simulink model "Trabalho1_Jesse_Beatriz_simulink"  (R2016a)
settings: Solver=VariableStepAuto  StartTime=0.0  StopTime=30  RelTol=1e-3
libraries: simulink x9
settings Model: Creator=jessa  LastModifiedBy=jessa

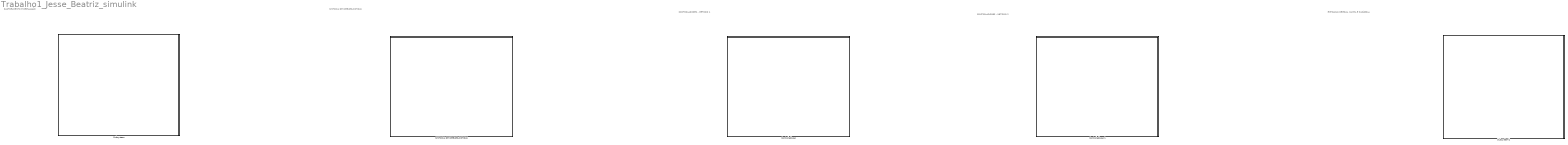
== system Trabalho1_Jesse_Beatriz_simulink ==
  note: CONTROLADORES - METODO 1
  note: SINTONIA DE ZIEGLER-NICHOLS
  note: CONTROLADORES - METODO 2
  note: RASTREAMENTO E REGULAÇÃO
  note: ENTRADAS DEGRAU, RAMPA E PARÁBOLA
  "Controladores " : Subsystem
  Controladores 1 : Subsystem
  SINTONIA DE ZIEGLER-NICHOLS : Subsystem
  Subsystem : Subsystem
  Subsystem1 : Subsystem

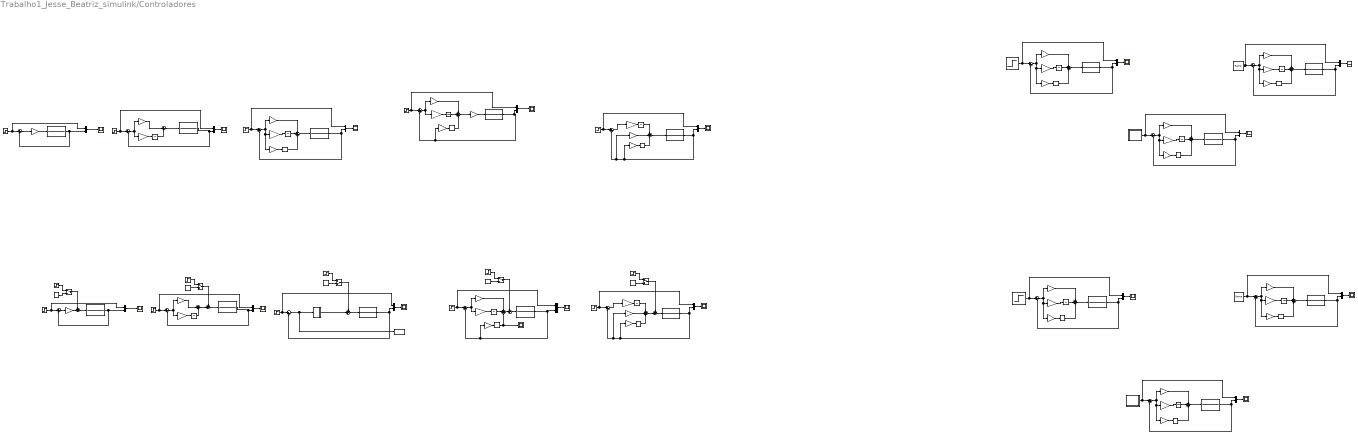
== system Trabalho1_Jesse_Beatriz_simulink/Controladores  ==
  note: E(s)
  note: U(s)
  note: PROPORCIONAL (P)
  note: PROPORCIONAL - INTEGRAL (PI)
  note: PROPORCIONAL - INTEGRAL - DERIVATIVO (PID)
  note: METODO 1
  note: PROPORCIONAL (P)
  note: PROPORCIONAL - INTEGRAL (PI)
  note: PROPORCIONAL - INTEGRAL - DERIVATIVO (PID)
  note: Controlador Sintonizado
  note: E(s)
  note: E(s)
  note: U(s)
  note: PI-D
  note: I-PD
  note: E(s)
  note: E(s)
  note: PI-D
  note: I-PD
  note: DEGRAU
  note: RAMPA
  note: PARABOLA
  note: ENTRADAS DEGRAU, RAMPA E PARÁBOLA
  note: E(s)
  note: U(s)
  note: E(s)
  note: U(s)
  note: E(s)
  note: U(s)
  note: E(s)
  note: U(s)
  note: E(s)
  note: U(s)
  note: E(s)
  note: U(s)
  note: DEGRAU
  note: RAMPA
  note: PARABOLA
  Constant{,1..4} (5 alike) : Constant  Value=0
  Derivative{,2..11} (11 alike) : Derivative
  Entrada Parabola Unitaria : Subsystem
  Entrada Parabola Unitaria1 : Subsystem
  Gain : Gain  Gain=8.0185
  Gain1 : Gain  Gain=6
  Integrator{,1..2,4..13} (13 alike) : Integrator
  Ki : Gain  Gain=10.8304
  Ki{1,8,14,16,18} (5 alike) : Gain  Gain=24.0676
  Ki{10,20,22,24} (4 alike) : Gain  Gain=5
  Ki{3,11,13,21,23,25} (6 alike) : Gain  Gain=2
  Ki12 : Gain  Gain=9
  Ki{2,9,15,17,19} (5 alike) : Gain  Gain=0.9617
  Ki6 : Gain  Gain=2.5013
  Ki7 : Gain  Gain=0.099
  Kp : Gain  Gain=7.2167
  Kp{1,5,8..11} (6 alike) : Gain  Gain=9.6222
  Kp{6,12..14} (4 alike) : Gain  Gain=12
  Kp2 : Gain  Gain=4
  Kp4 : Gain
  Kp7 : Gain  Gain=5
  Manual Switch{,1,3..4} (4 alike) : ManualSwitch
  Manual Switch2 : ManualSwitch  CurrentSetting=0
  Mux{1..16} (16 alike) : Mux  Inputs=2
  PID_Sintonizado : Subsystem
  Ramp : simulink/Sources/Ramp  slope=1  start=0  X0=0
  Ramp1 : simulink/Sources/Ramp  slope=1  start=0  X0=0
  Scope{1..16,18} (17 alike) : Scope
  Step{1..2,4..5,7..8,10..11,15} (9 alike) : Step  Time=0  SampleTime=0
  Step{12..14,16..17} (5 alike) : Step  Time=10  After=-1  SampleTime=0
  Step3 : Step  SampleTime=0
  Step6 : Step  SampleTime=0
  Step9 : Step  SampleTime=0
  Sum{1..2,4,6..7,9,11,13,15,17,19,21,23,26,28,30} (16 alike) : Sum  Inputs=|+-
  Sum12 : Sum  Inputs=++-
  Sum14 : Sum  Inputs=+--
  Sum16 : Sum  Inputs=++-
  Sum18 : Sum  Inputs=+--
  Sum{5,20,22,24..25,27,29} (7 alike) : Sum  Inputs=+++
  Sum3 : Sum  Inputs=|++
  Sum{31..35} (5 alike) : Sum  Inputs=++|
  Sum8 : Sum  Inputs=|++
  To Workspace : ToWorkspace  VariableName=Erro_PID  SampleTime=-1
  Transfer Fcn{1..16} (16 alike) : TransferFcn  Numerator=[45]  Denominator=[1 15 59 45]
  wires:
  Sum1/1 -> Gain/1
  Mux1/1 -> Scope1/1
  Transfer Fcn1/1 -> Sum1/2, Mux1/2
  Step1/1 -> Sum1/1, Mux1/1
  Gain/1 -> Transfer Fcn1/1
  Sum2/1 -> Ki/1, Kp/1
  Mux2/1 -> Scope2/1
  Transfer Fcn2/1 -> Mux2/2, Sum2/2
  Step2/1 -> Sum2/1, Mux2/1
  Kp/1 -> Sum3/1
  Sum3/1 -> Transfer Fcn2/1
  Ki/1 -> Integrator/1
  Integrator/1 -> Sum3/2
  Sum4/1 -> Kp1/1, Ki2/1, Ki1/1
  Mux3/1 -> Scope3/1
  Transfer Fcn3/1 -> Mux3/2, Sum4/2
  Step3/1 -> Mux3/1, Sum4/1
  Kp1/1 -> Sum5/1
  Sum5/1 -> Transfer Fcn3/1
  Ki1/1 -> Integrator1/1
  Integrator1/1 -> Sum5/2
  Ki2/1 -> Derivative/1
  Derivative/1 -> Sum5/3
  Sum6/1 -> Gain1/1
  Mux4/1 -> Scope4/1
  Transfer Fcn4/1 -> Mux4/2, Sum6/2
  Step4/1 -> Mux4/1, Sum6/1
  Sum7/1 -> Kp2/1, Ki3/1
  Mux5/1 -> Scope5/1
  Transfer Fcn5/1 -> Sum7/2, Mux5/2
  Step5/1 -> Mux5/1, Sum7/1
  Kp2/1 -> Sum8/1
  Ki3/1 -> Integrator2/1
  Integrator2/1 -> Sum8/2
  Mux6/1 -> Scope6/1
  Transfer Fcn6/1 -> Sum9/2, Mux6/2
  Step6/1 -> Mux6/1, Sum9/1
  Sum11/1 -> Ki6/1, Kp4/1
  Mux7/1 -> Scope7/1
  Transfer Fcn7/1 -> Ki7/1, Sum11/2, Mux7/2
  Step7/1 -> Sum11/1, Mux7/1
  Kp4/1 -> Sum12/1
  Ki6/1 -> Integrator4/1
  Integrator4/1 -> Sum12/2
  Ki7/1 -> Derivative2/1
  Derivative2/1 -> Sum12/3
  Sum13/1 -> Ki8/1
  Mux8/1 -> Scope8/1
  Transfer Fcn8/1 -> Mux8/2, Ki9/1, Kp5/1, Sum13/2
  Step8/1 -> Mux8/1, Sum13/1
  Sum14/1 -> Transfer Fcn8/1
  Ki8/1 -> Integrator5/1
  Ki9/1 -> Derivative3/1
  Derivative3/1 -> Sum14/3
  Kp5/1 -> Sum14/2
  Integrator5/1 -> Sum14/1
  Sum15/1 -> Kp6/1, Ki10/1
  Mux9/1 -> Scope9/1
  Transfer Fcn9/1 -> Mux9/2, Sum15/2, Ki11/1
  Step9/1 -> Mux9/1, Sum15/1
  Kp6/1 -> Sum16/1
  Ki10/1 -> Integrator6/1
  Integrator6/1 -> Sum16/2
  Ki11/1 -> Derivative4/1
  Sum17/1 -> Ki12/1
  Mux10/1 -> Scope10/1
  Transfer Fcn10/1 -> Sum17/2, Kp7/1, Ki13/1, Mux10/2
  Step10/1 -> Sum17/1, Mux10/1
  Ki12/1 -> Integrator7/1
  Ki13/1 -> Derivative5/1
  Derivative5/1 -> Sum18/3
  Kp7/1 -> Sum18/2
  Integrator7/1 -> Sum18/1
  Kp8/1 -> Transfer Fcn7/1
  Sum12/1 -> Kp8/1
  Sum19/1 -> Kp9/1, Ki15/1, Ki14/1
  Mux11/1 -> Scope11/1
  Transfer Fcn11/1 -> Mux11/2, Sum19/2
  Step11/1 -> Mux11/1, Sum19/1
  Kp9/1 -> Sum20/1
  Sum20/1 -> Transfer Fcn11/1
  Ki14/1 -> Integrator8/1
  Integrator8/1 -> Sum20/2
  Ki15/1 -> Derivative6/1
  Derivative6/1 -> Sum20/3
  Sum21/1 -> Kp10/1, Ki17/1, Ki16/1
  Mux12/1 -> Scope12/1
  Transfer Fcn12/1 -> Mux12/2, Sum21/2
  Entrada Parabola Unitaria/1(Out1) -> Mux12/1, Sum21/1
  Kp10/1 -> Sum22/1
  Sum22/1 -> Transfer Fcn12/1
  Ki16/1 -> Integrator9/1
  Integrator9/1 -> Sum22/2
  Ki17/1 -> Derivative7/1
  Derivative7/1 -> Sum22/3
  Sum23/1 -> Kp11/1, Ki19/1, Ki18/1
  Mux13/1 -> Scope13/1
  Transfer Fcn13/1 -> Mux13/2, Sum23/2
  Ramp/1 -> Mux13/1, Sum23/1
  Kp11/1 -> Sum24/1
  Sum24/1 -> Transfer Fcn13/1
  Ki18/1 -> Integrator10/1
  Integrator10/1 -> Sum24/2
  Ki19/1 -> Derivative8/1
  Derivative8/1 -> Sum24/3
  Sum26/1 -> Ki20/1, Ki21/1, Kp12/1
  Mux14/1 -> Scope14/1
  Transfer Fcn14/1 -> Sum26/2, Mux14/2
  Step15/1 -> Sum26/1, Mux14/1
  Kp12/1 -> Sum25/1
  Sum25/1 -> Transfer Fcn14/1
  Ki20/1 -> Integrator11/1
  Integrator11/1 -> Sum25/2
  Ki21/1 -> Derivative9/1
  Derivative9/1 -> Sum25/3
  Sum28/1 -> Ki23/1, Ki22/1, Kp13/1
  Mux15/1 -> Scope15/1
  Transfer Fcn15/1 -> Sum28/2, Mux15/2
  Ramp1/1 -> Sum28/1, Mux15/1
  Kp13/1 -> Sum27/1
  Sum27/1 -> Transfer Fcn15/1
  Ki22/1 -> Integrator12/1
  Integrator12/1 -> Sum27/2
  Ki23/1 -> Derivative10/1
  Derivative10/1 -> Sum27/3
  Sum30/1 -> Ki24/1, Ki25/1, Kp14/1
  Mux16/1 -> Scope16/1
  Transfer Fcn16/1 -> Sum30/2, Mux16/2
  Entrada Parabola Unitaria1/1(Out1) -> Sum30/1, Mux16/1
  Kp14/1 -> Sum29/1
  Sum29/1 -> Transfer Fcn16/1
  Ki24/1 -> Integrator13/1
  Integrator13/1 -> Sum29/2
  Ki25/1 -> Derivative11/1
  Derivative11/1 -> Sum29/3
  Gain1/1 -> Sum31/2
  Sum31/1 -> Transfer Fcn4/1
  Step12/1 -> Manual Switch/1
  Manual Switch/1 -> Sum31/1
  Step13/1 -> Manual Switch1/1
  Manual Switch1/1 -> Sum32/1
  Sum8/1 -> Sum32/2
  Sum32/1 -> Transfer Fcn5/1
  Step14/1 -> Manual Switch2/1
  Manual Switch2/1 -> Sum33/1
  Sum33/1 -> Transfer Fcn6/1
  Step16/1 -> Manual Switch3/1
  Manual Switch3/1 -> Sum34/1
  Step17/1 -> Manual Switch4/1
  Manual Switch4/1 -> Sum35/1
  Sum16/1 -> Sum34/2
  Sum34/1 -> Transfer Fcn9/1
  Sum18/1 -> Sum35/2
  Sum35/1 -> Transfer Fcn10/1
  Constant/1 -> Manual Switch/2
  Constant1/1 -> Manual Switch1/2
  Constant2/1 -> Manual Switch2/2
  Constant3/1 -> Manual Switch3/2
  Constant4/1 -> Manual Switch4/2
  Derivative4/1 -> Scope18/1, Sum16/3
  PID_Sintonizado/1(Out1) -> Sum33/2
  Sum9/1 -> To Workspace/1, PID_Sintonizado/1(In1)

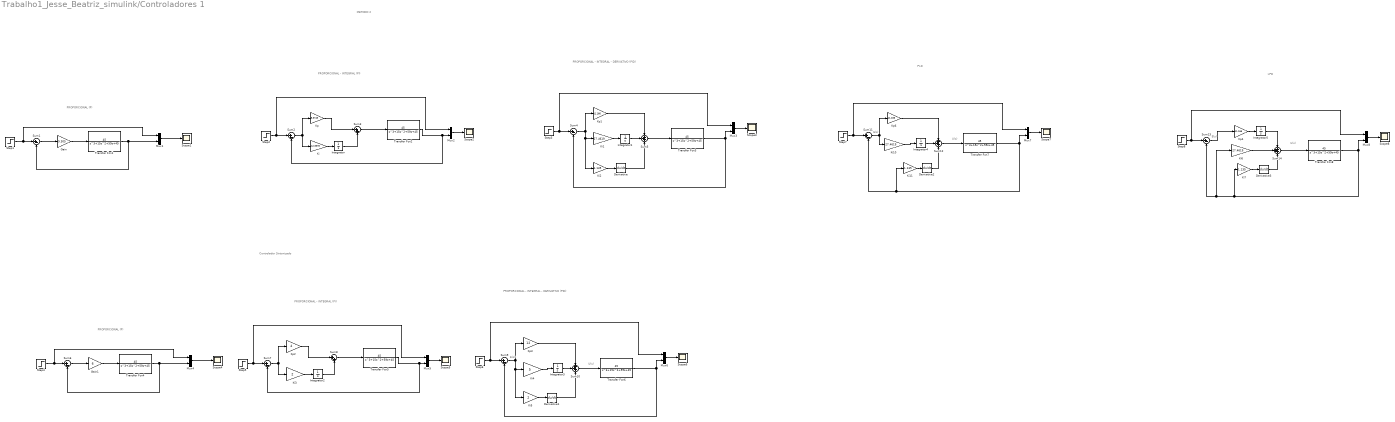
== system Trabalho1_Jesse_Beatriz_simulink/Controladores 1 ==
  note: PROPORCIONAL - INTEGRAL - DERIVATIVO (PID)
  note: PROPORCIONAL - INTEGRAL (PI)
  note: PROPORCIONAL (P)
  note: E(s)
  note: U(s)
  note: PROPORCIONAL (P)
  note: PROPORCIONAL - INTEGRAL (PI)
  note: PROPORCIONAL - INTEGRAL - DERIVATIVO (PID)
  note: Controlador Sintonizado
  note: METODO 2
  note: E(s)
  note: U(s)
  note: E(s)
  note: U(s)
  note: PI-D
  note: I-PD
  Derivative{,1..3} (4 alike) : Derivative
  Gain : Gain  Gain=9.305
  Gain1 : Gain  Gain=6
  Integrator{,1..5} (6 alike) : Integrator
  Ki : Gain  Gain=12.3578
  Ki1 : Gain  Gain=27.4619
  Ki10 : Gain  Gain=27.4619
  Ki11 : Gain  Gain=1.135
  Ki2 : Gain  Gain=1.135
  Ki3 : Gain  Gain=2
  Ki4 : Gain  Gain=5
  Ki5 : Gain  Gain=2
  Ki6 : Gain  Gain=27.4619
  Ki7 : Gain  Gain=1.135
  Kp : Gain  Gain=8.3745
  Kp1 : Gain  Gain=11.166
  Kp2 : Gain  Gain=4
  Kp3 : Gain  Gain=12
  Kp4 : Gain  Gain=11.166
  Kp6 : Gain  Gain=11.166
  Mux{1..8} (8 alike) : Mux  Inputs=2
  Scope{1..8} (8 alike) : Scope
  Step{1..8} (8 alike) : Step  Time=0  SampleTime=0
  Sum{1..2,4,6..7,9,11,13} (8 alike) : Sum  Inputs=|+-
  Sum{5,10,12,14} (4 alike) : Sum  Inputs=+++
  Sum3 : Sum  Inputs=|++
  Sum8 : Sum  Inputs=|++
  Transfer Fcn{1..8} (8 alike) : TransferFcn  Numerator=[45]  Denominator=[1 15 59 45]
  wires:
  Derivative/1 -> Sum5/3
  Ki2/1 -> Derivative/1
  Integrator1/1 -> Sum5/2
  Ki1/1 -> Integrator1/1
  Sum5/1 -> Transfer Fcn3/1
  Kp1/1 -> Sum5/1
  Step3/1 -> Sum4/1, Mux3/1
  Transfer Fcn3/1 -> Sum4/2, Mux3/2
  Mux3/1 -> Scope3/1
  Sum4/1 -> Ki1/1, Ki2/1, Kp1/1
  Integrator/1 -> Sum3/2
  Ki/1 -> Integrator/1
  Sum3/1 -> Transfer Fcn2/1
  Kp/1 -> Sum3/1
  Step2/1 -> Mux2/1, Sum2/1
  Transfer Fcn2/1 -> Sum2/2, Mux2/2
  Mux2/1 -> Scope2/1
  Sum2/1 -> Kp/1, Ki/1
  Gain/1 -> Transfer Fcn1/1
  Step1/1 -> Mux1/1, Sum1/1
  Transfer Fcn1/1 -> Mux1/2, Sum1/2
  Mux1/1 -> Scope1/1
  Sum1/1 -> Gain/1
  Sum6/1 -> Gain1/1
  Mux4/1 -> Scope4/1
  Transfer Fcn4/1 -> Mux4/2, Sum6/2
  Step4/1 -> Mux4/1, Sum6/1
  Gain1/1 -> Transfer Fcn4/1
  Sum7/1 -> Kp2/1, Ki3/1
  Mux5/1 -> Scope5/1
  Transfer Fcn5/1 -> Sum7/2, Mux5/2
  Step5/1 -> Mux5/1, Sum7/1
  Kp2/1 -> Sum8/1
  Sum8/1 -> Transfer Fcn5/1
  Ki3/1 -> Integrator2/1
  Integrator2/1 -> Sum8/2
  Sum9/1 -> Ki4/1, Ki5/1, Kp3/1
  Mux6/1 -> Scope6/1
  Transfer Fcn6/1 -> Sum9/2, Mux6/2
  Step6/1 -> Sum9/1, Mux6/1
  Kp3/1 -> Sum10/1
  Sum10/1 -> Transfer Fcn6/1
  Ki4/1 -> Integrator3/1
  Integrator3/1 -> Sum10/2
  Ki5/1 -> Derivative1/1
  Derivative1/1 -> Sum10/3
  Sum11/1 -> Ki10/1, Kp6/1
  Mux7/1 -> Scope7/1
  Transfer Fcn7/1 -> Ki11/1, Sum11/2, Mux7/2
  Step7/1 -> Sum11/1, Mux7/1
  Kp6/1 -> Sum12/1
  Sum12/1 -> Transfer Fcn7/1
  Ki10/1 -> Integrator4/1
  Integrator4/1 -> Sum12/2
  Ki11/1 -> Derivative2/1
  Derivative2/1 -> Sum12/3
  Sum13/1 -> Kp4/1
  Mux8/1 -> Scope8/1
  Transfer Fcn8/1 -> Mux8/2, Ki7/1, Ki6/1, Sum13/2
  Step8/1 -> Mux8/1, Sum13/1
  Sum14/1 -> Transfer Fcn8/1
  Kp4/1 -> Integrator5/1
  Ki7/1 -> Derivative3/1
  Derivative3/1 -> Sum14/3
  Ki6/1 -> Sum14/2
  Integrator5/1 -> Sum14/1

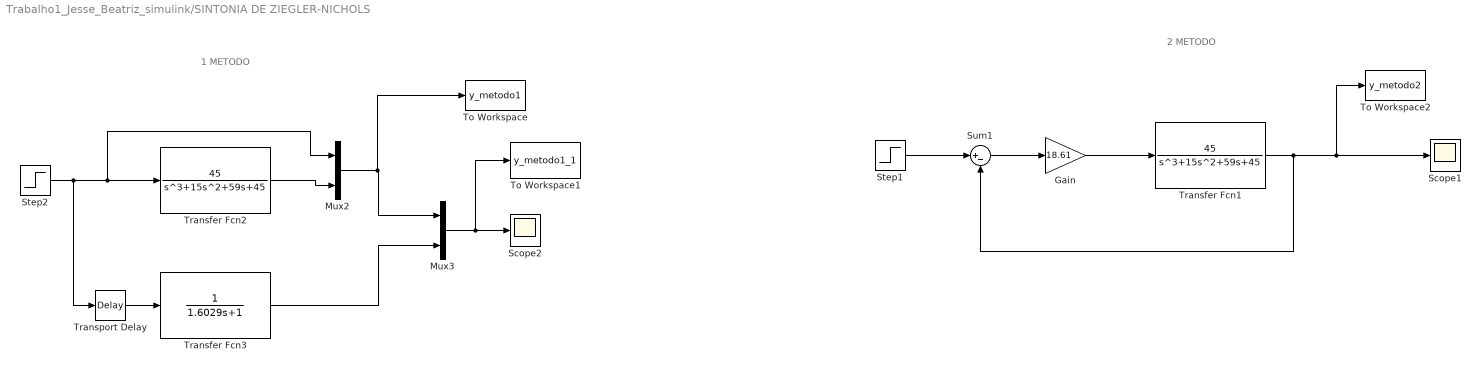
== system Trabalho1_Jesse_Beatriz_simulink/SINTONIA DE ZIEGLER-NICHOLS ==
  note: 1 METODO
  note: 2 METODO
  Gain : Gain  Gain=18.61
  Mux2 : Mux  Inputs=2
  Mux3 : Mux  Inputs=2
  Scope1 : Scope
  Scope2 : Scope
  Step1 : Step  Time=0  SampleTime=0
  Step2 : Step  Time=0  SampleTime=0
  Sum1 : Sum  Inputs=|+-
  To Workspace : ToWorkspace  VariableName=y_metodo1  SampleTime=-1
  To Workspace1 : ToWorkspace  VariableName=y_metodo1_1  SampleTime=-1
  To Workspace2 : ToWorkspace  VariableName=y_metodo2  SampleTime=-1
  Transfer Fcn1 : TransferFcn  Numerator=[45]  Denominator=[1 15 59 45]
  Transfer Fcn2 : TransferFcn  Numerator=[45]  Denominator=[1 15 59 45]
  Transfer Fcn3 : TransferFcn  Denominator=[1.6029 1]
  Transport Delay : TransportDelay  DelayTime=0.1999
  wires:
  Gain/1 -> Transfer Fcn1/1
  Step1/1 -> Sum1/1
  Transfer Fcn1/1 -> To Workspace2/1, Scope1/1, Sum1/2
  Sum1/1 -> Gain/1
  Step2/1 -> Transport Delay/1, Transfer Fcn2/1, Mux2/1
  Transfer Fcn2/1 -> Mux2/2
  Transport Delay/1 -> Transfer Fcn3/1
  Mux2/1 -> To Workspace/1, Mux3/1
  Transfer Fcn3/1 -> Mux3/2
  Mux3/1 -> To Workspace1/1, Scope2/1

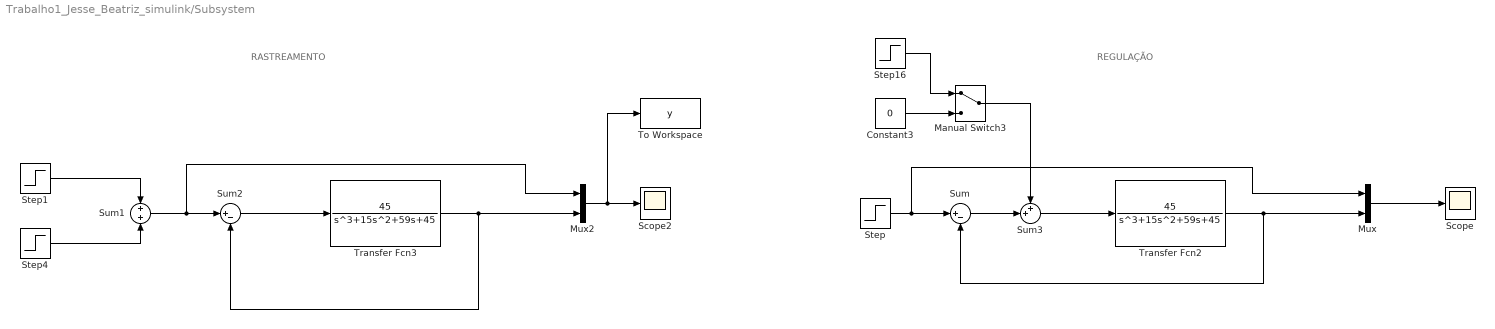
== system Trabalho1_Jesse_Beatriz_simulink/Subsystem ==
  note: REGULAÇÃO
  note: RASTREAMENTO
  Constant3 : Constant  Value=0
  Manual Switch3 : ManualSwitch
  Mux : Mux  Inputs=2
  Mux2 : Mux  Inputs=2
  Scope : Scope
  Scope2 : Scope
  Step : Step  Time=0  After=2  SampleTime=0
  Step1 : Step  Time=0  SampleTime=0
  Step16 : Step  Time=10  After=-1  SampleTime=0
  Step4 : Step  Time=15  After=3  SampleTime=0
  Sum : Sum  Inputs=|+-
  Sum1 : Sum  Inputs=+|+
  Sum2 : Sum  Inputs=|+-
  Sum3 : Sum  Inputs=++|
  To Workspace : ToWorkspace  VariableName=y  SampleTime=-1
  Transfer Fcn2 : TransferFcn  Numerator=[45]  Denominator=[1 15 59 45]
  Transfer Fcn3 : TransferFcn  Numerator=[45]  Denominator=[1 15 59 45]
  wires:
  Step/1 -> Sum/1, Mux/1
  Mux2/1 -> To Workspace/1, Scope2/1
  Sum1/1 -> Sum2/1, Mux2/1
  Mux/1 -> Scope/1
  Transfer Fcn2/1 -> Mux/2, Sum/2
  Transfer Fcn3/1 -> Sum2/2, Mux2/2
  Sum2/1 -> Transfer Fcn3/1
  Step1/1 -> Sum1/1
  Step4/1 -> Sum1/2
  Sum/1 -> Sum3/2
  Sum3/1 -> Transfer Fcn2/1
  Manual Switch3/1 -> Sum3/1
  Step16/1 -> Manual Switch3/1
  Constant3/1 -> Manual Switch3/2

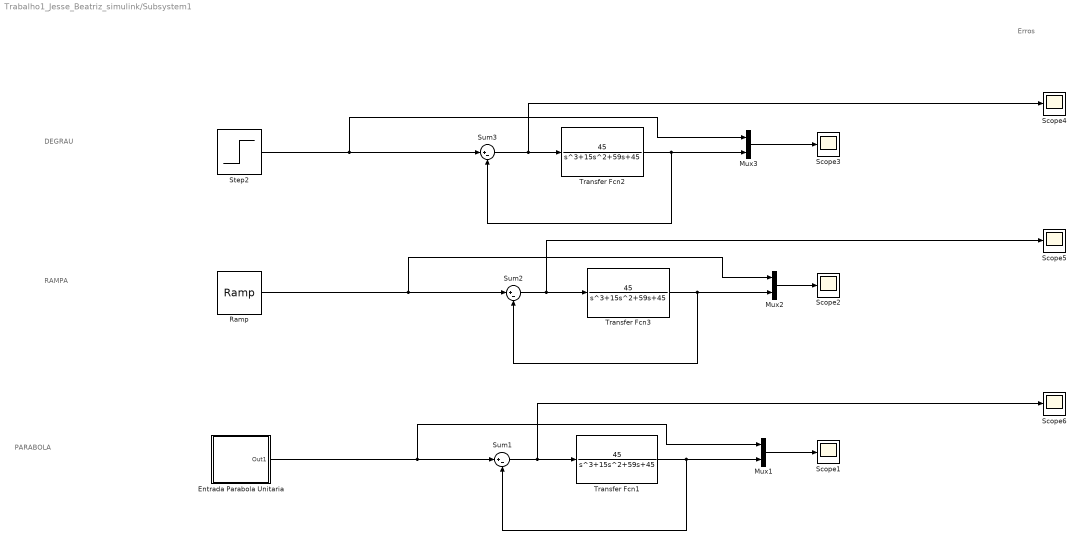
== system Trabalho1_Jesse_Beatriz_simulink/Subsystem1 ==
  note: DEGRAU
  note: RAMPA
  note: PARABOLA
  note: Erros
  Entrada Parabola Unitaria : Subsystem
  Mux1 : Mux  Inputs=2
  Mux2 : Mux  Inputs=2
  Mux3 : Mux  Inputs=2
  Ramp : simulink/Sources/Ramp  slope=1  start=0  X0=0
  Scope{1..6} (6 alike) : Scope
  Step2 : Step  Time=0  SampleTime=0
  Sum1 : Sum  Inputs=|+-
  Sum2 : Sum  Inputs=|+-
  Sum3 : Sum  Inputs=|+-
  Transfer Fcn1 : TransferFcn  Numerator=[45]  Denominator=[1 15 59 45]
  Transfer Fcn2 : TransferFcn  Numerator=[45]  Denominator=[1 15 59 45]
  Transfer Fcn3 : TransferFcn  Numerator=[45]  Denominator=[1 15 59 45]
  wires:
  Entrada Parabola Unitaria/1(Out1) -> Mux1/1, Sum1/1
  Ramp/1 -> Mux2/1, Sum2/1
  Mux2/1 -> Scope2/1
  Transfer Fcn3/1 -> Sum2/2, Mux2/2
  Sum2/1 -> Scope5/1, Transfer Fcn3/1
  Mux1/1 -> Scope1/1
  Transfer Fcn1/1 -> Mux1/2, Sum1/2
  Sum1/1 -> Scope6/1, Transfer Fcn1/1
  Mux3/1 -> Scope3/1
  Transfer Fcn2/1 -> Sum3/2, Mux3/2
  Sum3/1 -> Scope4/1, Transfer Fcn2/1
  Step2/1 -> Mux3/1, Sum3/1

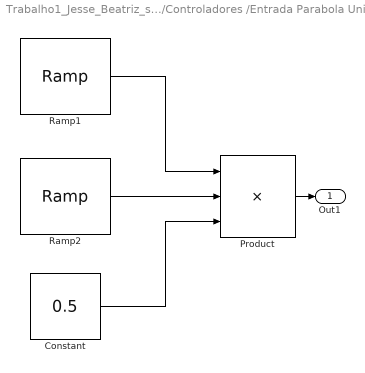
== system Trabalho1_Jesse_Beatriz_simulink/Controladores /Entrada Parabola Unitaria ==
  Constant : Constant  Value=0.5
  Product : Product  Inputs=3
  Ramp1 : simulink/Sources/Ramp  slope=1  start=0  X0=0
  Ramp2 : simulink/Sources/Ramp  slope=1  start=0  X0=0
  Out1 : Outport
  wires:
  Ramp2/1 -> Product/2
  Constant/1 -> Product/3
  Product/1 -> Out1/1
  Ramp1/1 -> Product/1

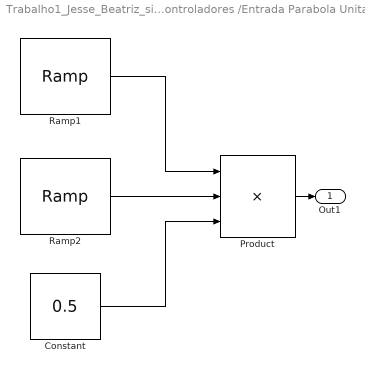
== system Trabalho1_Jesse_Beatriz_simulink/Controladores /Entrada Parabola Unitaria1 ==
  Constant : Constant  Value=0.5
  Product : Product  Inputs=3
  Ramp1 : simulink/Sources/Ramp  slope=1  start=0  X0=0
  Ramp2 : simulink/Sources/Ramp  slope=1  start=0  X0=0
  Out1 : Outport
  wires:
  Ramp2/1 -> Product/2
  Constant/1 -> Product/3
  Product/1 -> Out1/1
  Ramp1/1 -> Product/1

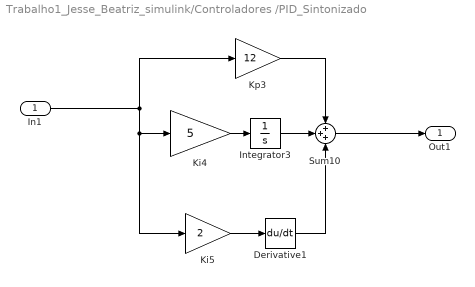
== system Trabalho1_Jesse_Beatriz_simulink/Controladores /PID_Sintonizado ==
  In1 : Inport
  Derivative1 : Derivative
  Integrator3 : Integrator
  Ki4 : Gain  Gain=5
  Ki5 : Gain  Gain=2
  Kp3 : Gain  Gain=12
  Sum10 : Sum  Inputs=+++
  Out1 : Outport
  wires:
  Ki4/1 -> Integrator3/1
  Ki5/1 -> Derivative1/1
  In1/1 -> Ki5/1, Ki4/1, Kp3/1
  Kp3/1 -> Sum10/1
  Derivative1/1 -> Sum10/3
  Integrator3/1 -> Sum10/2
  Sum10/1 -> Out1/1

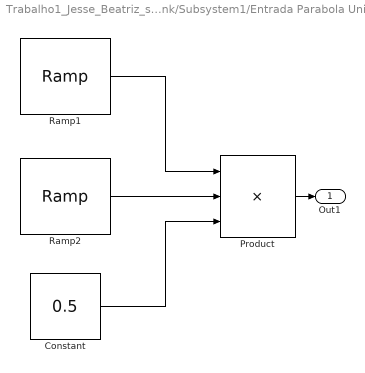
== system Trabalho1_Jesse_Beatriz_simulink/Subsystem1/Entrada Parabola Unitaria ==
  Constant : Constant  Value=0.5
  Product : Product  Inputs=3
  Ramp1 : simulink/Sources/Ramp  slope=1  start=0  X0=0
  Ramp2 : simulink/Sources/Ramp  slope=1  start=0  X0=0
  Out1 : Outport
  wires:
  Ramp2/1 -> Product/2
  Constant/1 -> Product/3
  Product/1 -> Out1/1
  Ramp1/1 -> Product/1
